simulink model "UnitDelayBlock1"  (R2023a)
settings: Solver=VariableStepAuto  StartTime=0.0  StopTime=10.0  RelTol=1e-3
settings Model: Creator=aan18022  LastModifiedBy=aan18022

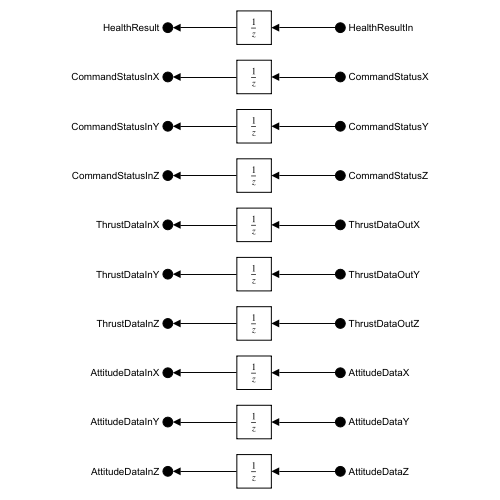
[thumbnail: Simulink's stored preview of the top-level diagram]
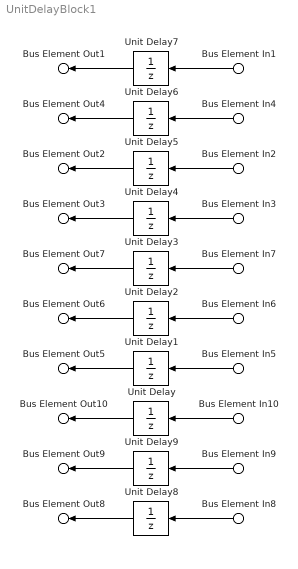
== system UnitDelayBlock1 ==
  Bus Element In9 : Inport  PortName=AttitudeDataY
  Bus Element In5 : Inport  Port=2  PortName=ThrustDataOutZ
  Bus Element In1 : Inport  Port=3  PortName=HealthResultIn
  Bus Element In2 : Inport  Port=4  PortName=CommandStatusY
  Bus Element In3 : Inport  Port=5  PortName=CommandStatusZ
  Bus Element In4 : Inport  Port=6  PortName=CommandStatusX
  Bus Element In6 : Inport  Port=7  PortName=ThrustDataOutY
  Bus Element In7 : Inport  Port=8  PortName=ThrustDataOutX
  Bus Element In8 : Inport  Port=9  PortName=AttitudeDataZ
  Bus Element In10 : Inport  Port=10  PortName=AttitudeDataX
  Unit Delay{,1..9} (10 alike) : UnitDelay  SampleTime=-1  HasFrameUpgradeWarning=on
  Bus Element Out1 : Outport  PortName=HealthResult
  Bus Element Out2 : Outport  Port=2  PortName=CommandStatusInY
  Bus Element Out3 : Outport  Port=3  PortName=CommandStatusInZ
  Bus Element Out4 : Outport  Port=4  PortName=CommandStatusInX
  Bus Element Out5 : Outport  Port=5  PortName=ThrustDataInZ
  Bus Element Out6 : Outport  Port=6  PortName=ThrustDataInY
  Bus Element Out7 : Outport  Port=7  PortName=ThrustDataInX
  Bus Element Out8 : Outport  Port=8  PortName=AttitudeDataInZ
  Bus Element Out9 : Outport  Port=9  PortName=AttitudeDataInY
  Bus Element Out10 : Outport  Port=10  PortName=AttitudeDataInX
  wires:
  Bus Element In1/1 -> Unit Delay7/1
  Bus Element In4/1 -> Unit Delay6/1
  Bus Element In2/1 -> Unit Delay5/1
  Bus Element In3/1 -> Unit Delay4/1
  Bus Element In7/1 -> Unit Delay3/1
  Bus Element In6/1 -> Unit Delay2/1
  Bus Element In5/1 -> Unit Delay1/1
  Bus Element In10/1 -> Unit Delay/1
  Bus Element In9/1 -> Unit Delay9/1
  Bus Element In8/1 -> Unit Delay8/1
  Unit Delay7/1 -> Bus Element Out1/1
  Unit Delay6/1 -> Bus Element Out4/1
  Unit Delay5/1 -> Bus Element Out2/1
  Unit Delay4/1 -> Bus Element Out3/1
  Unit Delay3/1 -> Bus Element Out7/1
  Unit Delay2/1 -> Bus Element Out6/1
  Unit Delay1/1 -> Bus Element Out5/1
  Unit Delay/1 -> Bus Element Out10/1
  Unit Delay9/1 -> Bus Element Out9/1
  Unit Delay8/1 -> Bus Element Out8/1
